simulink library "AEMS_Standard_Library"  (R2016b)
settings: Solver=ode45  StartTime=0.0  StopTime=10.0  RelTol=1e-3
undefined symbols (not defined in the file or in its folder): BkPY, carto, Cbx_extegr, Cbx_lpegrsys, Cbx_portegr, Cnx_bnk_nr_conf, Cnx_cyl_nr_conf, ConfigManagement, configuration_management, Cxx_dcm_io_tmr_end_xxxx, Cxx_dcm_rt_tmr_end, Cxx_DID_xxxx_IO_max, Cxx_DID_xxxx_IO_min, Cxx_egrhsofs, Cxx_vmaniegi, DEM_DEBOUNCE_FREEZE, DEM_DTR_CTL_INVISIBLE, DEM_DTR_CTL_NORMAL, Dem_DtrId2_XXX, Dem_DtrId3_XXX, Dem_DtrId4_XXX, Dem_DtrId5_XXX, Dem_DtrId6_XXX, Dem_DtrId7_XXX, Dem_DtrId8_XXX, Dem_DtrId9_XXX, Dem_DtrId_XXX, Dem_EnableConditionId2_XXX, Dem_EnableConditionId3_XXX, Dem_EnableConditionId4_XXX, Dem_EnableConditionId5_XXX, Dem_EnableConditionId6_XXX, Dem_EnableConditionId7_XXX, Dem_EnableConditionId8_XXX, Dem_EnableConditionId_XXX, Dem_EventId, Dem_EventId2_XXX, Dem_EventId3_XXX, Dem_EventId4_XXX, Dem_EventId5_XXX, Dem_EventId6_XXX, Dem_EventId7_XXX, Dem_EventId8_XXX, Dem_EventId9_XXX, Dem_EventId_Device_Faulttype, Dem_EventId_XXX, DEM_IUMPR_GENERAL_DENOMINATOR, DEM_OPCYC_IGNITION, Dem_RatioId2_XXX, Dem_RatioId3_XXX, Dem_RatioId4_XXX, Dem_RatioId5_XXX, Dem_RatioId6_XXX, Dem_RatioId7_XXX, Dem_RatioId8_XXX, Dem_RatioId_XXX, Dem_StorageConditionId2_XXX, Dem_StorageConditionId3_XXX, Dem_StorageConditionId4_XXX, Dem_StorageConditionId5_XXX ... (+65)
libraries: AEMS_Standard_Library x477, simulink x2
(part 22 of 39)

== system AEMS_Standard_Library/SUB/AEMS_DEM_COUNTER_BASED_DEBOUNCE_THRSHOLD_DYN_6D ==
  note: flag_set
  note: DemDebounceBehavior
  flag_set : Inport
  conditionfulfilled : Inport  Port=2
  prefailed : Inport  Port=3
  prepassed : Inport  Port=4
  failedthreshold : Inport  Port=5
  passedthreshold : Inport  Port=6
  reseteventdebounce : Inport  Port=7
  AEMS_DEM_COUNTER_BASED_DEBOUNCE_THRSHOLD_DYN_CALL1 : Subsystem
  AEMS_DEM_COUNTER_BASED_DEBOUNCE_THRSHOLD_DYN_CALL2 : Subsystem
  AEMS_DEM_COUNTER_BASED_DEBOUNCE_THRSHOLD_DYN_CALL3 : Subsystem
  AEMS_DEM_COUNTER_BASED_DEBOUNCE_THRSHOLD_DYN_CALL4 : Subsystem
  AEMS_DEM_COUNTER_BASED_DEBOUNCE_THRSHOLD_DYN_CALL5 : Subsystem
  AEMS_DEM_COUNTER_BASED_DEBOUNCE_THRSHOLD_DYN_CALL6 : Subsystem
  DemCounterDecrementStepSize : Constant  Value=DemCounterDecrementStepSize
  DemCounterIncrementStepSize : Constant  Value=DemCounterIncrementStepSize
  DemCounterJumpDown : Constant  Value=DemCounterJumpDown
  DemCounterJumpDownValue : Constant  Value=DemCounterJumpDownValue
  DemCounterJumpUp : Constant  Value=DemCounterJumpUp
  DemCounterJumpUpValue : Constant  Value=DemCounterJumpUpValue
  DemDebounceBehavior : Constant  Value=[0,0,0,0,0,0]  OutDataTypeStr=uint8
  Demux{,1..13} (14 alike) : Demux  Outputs=6
  Mux1 : Mux  Inputs=6
  Mux2 : Mux  Inputs=6
  Mux3 : Mux  Inputs=6
  debouncevalue : Outport
  failed : Outport  Port=2
  passed : Outport  Port=3
  wires:
  flag_set/1 -> Demux/1
  Demux/1 -> AEMS_DEM_COUNTER_BASED_DEBOUNCE_THRSHOLD_DYN_CALL1/Enable
  Demux/2 -> AEMS_DEM_COUNTER_BASED_DEBOUNCE_THRSHOLD_DYN_CALL2/Enable
  conditionfulfilled/1 -> Demux1/1  "conditionfulfilled"
  Demux1/1 -> AEMS_DEM_COUNTER_BASED_DEBOUNCE_THRSHOLD_DYN_CALL1/1(conditionfulfilled)
  Demux1/2 -> AEMS_DEM_COUNTER_BASED_DEBOUNCE_THRSHOLD_DYN_CALL2/1(conditionfulfilled)
  prefailed/1 -> Demux2/1  "prefailed"
  Demux2/1 -> AEMS_DEM_COUNTER_BASED_DEBOUNCE_THRSHOLD_DYN_CALL1/2(prefailed)
  Demux2/2 -> AEMS_DEM_COUNTER_BASED_DEBOUNCE_THRSHOLD_DYN_CALL2/2(prefailed)
  prepassed/1 -> Demux3/1  "prepassed"
  Demux3/1 -> AEMS_DEM_COUNTER_BASED_DEBOUNCE_THRSHOLD_DYN_CALL1/3(prepassed)
  Demux3/2 -> AEMS_DEM_COUNTER_BASED_DEBOUNCE_THRSHOLD_DYN_CALL2/3(prepassed)
  DemDebounceBehavior/1 -> Demux4/1  "behavior"
  Demux4/1 -> AEMS_DEM_COUNTER_BASED_DEBOUNCE_THRSHOLD_DYN_CALL1/4(DemDebounceBehavior)
  Demux4/2 -> AEMS_DEM_COUNTER_BASED_DEBOUNCE_THRSHOLD_DYN_CALL2/4(DemDebounceBehavior)
  failedthreshold/1 -> Demux5/1  "failedthreshold"
  Demux5/1 -> AEMS_DEM_COUNTER_BASED_DEBOUNCE_THRSHOLD_DYN_CALL1/5(failedthreshold)
  Demux5/2 -> AEMS_DEM_COUNTER_BASED_DEBOUNCE_THRSHOLD_DYN_CALL2/5(failedthreshold)
  DemCounterIncrementStepSize/1 -> Demux6/1  "incrementstepsize_for_prefailed"
  Demux6/1 -> AEMS_DEM_COUNTER_BASED_DEBOUNCE_THRSHOLD_DYN_CALL1/6(DemCounterIncrementStepSize)
  Demux6/2 -> AEMS_DEM_COUNTER_BASED_DEBOUNCE_THRSHOLD_DYN_CALL2/6(DemCounterIncrementStepSize)
  DemCounterJumpUp/1 -> Demux7/1  "jumpup_activation_with_prefailed"
  Demux7/1 -> AEMS_DEM_COUNTER_BASED_DEBOUNCE_THRSHOLD_DYN_CALL1/7(DemCounterJumpUp)
  Demux7/2 -> AEMS_DEM_COUNTER_BASED_DEBOUNCE_THRSHOLD_DYN_CALL2/7(DemCounterJumpUp)
  DemCounterJumpUpValue/1 -> Demux8/1  "jumpupvalue_with_prefailed"
  Demux8/1 -> AEMS_DEM_COUNTER_BASED_DEBOUNCE_THRSHOLD_DYN_CALL1/8(DemCounterJumpUpValue)
  Demux8/2 -> AEMS_DEM_COUNTER_BASED_DEBOUNCE_THRSHOLD_DYN_CALL2/8(DemCounterJumpUpValue)
  passedthreshold/1 -> Demux9/1  "passedthreshold"
  Demux9/1 -> AEMS_DEM_COUNTER_BASED_DEBOUNCE_THRSHOLD_DYN_CALL1/9(passedthreshold)
  Demux9/2 -> AEMS_DEM_COUNTER_BASED_DEBOUNCE_THRSHOLD_DYN_CALL2/9(passedthreshold)
  DemCounterDecrementStepSize/1 -> Demux10/1  "decrementstepsize_for_prepassed"
  Demux10/1 -> AEMS_DEM_COUNTER_BASED_DEBOUNCE_THRSHOLD_DYN_CALL1/10(DemCounterDecrementStepSize)
  Demux10/2 -> AEMS_DEM_COUNTER_BASED_DEBOUNCE_THRSHOLD_DYN_CALL2/10(DemCounterDecrementStepSize)
  DemCounterJumpDown/1 -> Demux11/1  "jumpdown_activation_with_prepassed"
  Demux11/1 -> AEMS_DEM_COUNTER_BASED_DEBOUNCE_THRSHOLD_DYN_CALL1/11(DemCounterJumpDown)
  Demux11/2 -> AEMS_DEM_COUNTER_BASED_DEBOUNCE_THRSHOLD_DYN_CALL2/11(DemCounterJumpDown)
  DemCounterJumpDownValue/1 -> Demux12/1  "jumpupvalue_with_prefailed"
  Demux12/1 -> AEMS_DEM_COUNTER_BASED_DEBOUNCE_THRSHOLD_DYN_CALL1/12(DemCounterJumpDownValue)
  Demux12/2 -> AEMS_DEM_COUNTER_BASED_DEBOUNCE_THRSHOLD_DYN_CALL2/12(DemCounterJumpDownValue)
  reseteventdebounce/1 -> Demux13/1  "reseteventdebounce"
  Demux13/1 -> AEMS_DEM_COUNTER_BASED_DEBOUNCE_THRSHOLD_DYN_CALL1/13(reseteventdebounce)
  Demux13/2 -> AEMS_DEM_COUNTER_BASED_DEBOUNCE_THRSHOLD_DYN_CALL2/13(reseteventdebounce)
  AEMS_DEM_COUNTER_BASED_DEBOUNCE_THRSHOLD_DYN_CALL1/1(debouncevalue) -> Mux1/1
  Mux1/1 -> debouncevalue/1
  AEMS_DEM_COUNTER_BASED_DEBOUNCE_THRSHOLD_DYN_CALL2/1(debouncevalue) -> Mux1/2
  AEMS_DEM_COUNTER_BASED_DEBOUNCE_THRSHOLD_DYN_CALL1/2(failed) -> Mux2/1
  Mux2/1 -> failed/1
  AEMS_DEM_COUNTER_BASED_DEBOUNCE_THRSHOLD_DYN_CALL2/2(failed) -> Mux2/2
  AEMS_DEM_COUNTER_BASED_DEBOUNCE_THRSHOLD_DYN_CALL1/3(passed) -> Mux3/1
  Mux3/1 -> passed/1
  AEMS_DEM_COUNTER_BASED_DEBOUNCE_THRSHOLD_DYN_CALL2/3(passed) -> Mux3/2
  Demux/3 -> AEMS_DEM_COUNTER_BASED_DEBOUNCE_THRSHOLD_DYN_CALL3/Enable
  Demux1/3 -> AEMS_DEM_COUNTER_BASED_DEBOUNCE_THRSHOLD_DYN_CALL3/1(conditionfulfilled)
  Demux2/3 -> AEMS_DEM_COUNTER_BASED_DEBOUNCE_THRSHOLD_DYN_CALL3/2(prefailed)
  Demux3/3 -> AEMS_DEM_COUNTER_BASED_DEBOUNCE_THRSHOLD_DYN_CALL3/3(prepassed)
  Demux4/3 -> AEMS_DEM_COUNTER_BASED_DEBOUNCE_THRSHOLD_DYN_CALL3/4(DemDebounceBehavior)
  Demux5/3 -> AEMS_DEM_COUNTER_BASED_DEBOUNCE_THRSHOLD_DYN_CALL3/5(failedthreshold)
  Demux6/3 -> AEMS_DEM_COUNTER_BASED_DEBOUNCE_THRSHOLD_DYN_CALL3/6(DemCounterIncrementStepSize)
  Demux7/3 -> AEMS_DEM_COUNTER_BASED_DEBOUNCE_THRSHOLD_DYN_CALL3/7(DemCounterJumpUp)
  Demux8/3 -> AEMS_DEM_COUNTER_BASED_DEBOUNCE_THRSHOLD_DYN_CALL3/8(DemCounterJumpUpValue)
  Demux9/3 -> AEMS_DEM_COUNTER_BASED_DEBOUNCE_THRSHOLD_DYN_CALL3/9(passedthreshold)
  Demux10/3 -> AEMS_DEM_COUNTER_BASED_DEBOUNCE_THRSHOLD_DYN_CALL3/10(DemCounterDecrementStepSize)
  Demux11/3 -> AEMS_DEM_COUNTER_BASED_DEBOUNCE_THRSHOLD_DYN_CALL3/11(DemCounterJumpDown)
  Demux12/3 -> AEMS_DEM_COUNTER_BASED_DEBOUNCE_THRSHOLD_DYN_CALL3/12(DemCounterJumpDownValue)
  Demux13/3 -> AEMS_DEM_COUNTER_BASED_DEBOUNCE_THRSHOLD_DYN_CALL3/13(reseteventdebounce)
  AEMS_DEM_COUNTER_BASED_DEBOUNCE_THRSHOLD_DYN_CALL3/1(debouncevalue) -> Mux1/3
  AEMS_DEM_COUNTER_BASED_DEBOUNCE_THRSHOLD_DYN_CALL3/2(failed) -> Mux2/3
  AEMS_DEM_COUNTER_BASED_DEBOUNCE_THRSHOLD_DYN_CALL3/3(passed) -> Mux3/3
  Demux/4 -> AEMS_DEM_COUNTER_BASED_DEBOUNCE_THRSHOLD_DYN_CALL4/Enable
  Demux/5 -> AEMS_DEM_COUNTER_BASED_DEBOUNCE_THRSHOLD_DYN_CALL5/Enable
  Demux/6 -> AEMS_DEM_COUNTER_BASED_DEBOUNCE_THRSHOLD_DYN_CALL6/Enable
  Demux1/4 -> AEMS_DEM_COUNTER_BASED_DEBOUNCE_THRSHOLD_DYN_CALL4/1(conditionfulfilled)
  Demux1/5 -> AEMS_DEM_COUNTER_BASED_DEBOUNCE_THRSHOLD_DYN_CALL5/1(conditionfulfilled)
  Demux1/6 -> AEMS_DEM_COUNTER_BASED_DEBOUNCE_THRSHOLD_DYN_CALL6/1(conditionfulfilled)
  Demux2/4 -> AEMS_DEM_COUNTER_BASED_DEBOUNCE_THRSHOLD_DYN_CALL4/2(prefailed)
  Demux2/5 -> AEMS_DEM_COUNTER_BASED_DEBOUNCE_THRSHOLD_DYN_CALL5/2(prefailed)
  Demux2/6 -> AEMS_DEM_COUNTER_BASED_DEBOUNCE_THRSHOLD_DYN_CALL6/2(prefailed)
  Demux3/4 -> AEMS_DEM_COUNTER_BASED_DEBOUNCE_THRSHOLD_DYN_CALL4/3(prepassed)
  Demux3/5 -> AEMS_DEM_COUNTER_BASED_DEBOUNCE_THRSHOLD_DYN_CALL5/3(prepassed)
  Demux3/6 -> AEMS_DEM_COUNTER_BASED_DEBOUNCE_THRSHOLD_DYN_CALL6/3(prepassed)
  Demux4/4 -> AEMS_DEM_COUNTER_BASED_DEBOUNCE_THRSHOLD_DYN_CALL4/4(DemDebounceBehavior)
  Demux4/5 -> AEMS_DEM_COUNTER_BASED_DEBOUNCE_THRSHOLD_DYN_CALL5/4(DemDebounceBehavior)
  Demux4/6 -> AEMS_DEM_COUNTER_BASED_DEBOUNCE_THRSHOLD_DYN_CALL6/4(DemDebounceBehavior)
  Demux5/4 -> AEMS_DEM_COUNTER_BASED_DEBOUNCE_THRSHOLD_DYN_CALL4/5(failedthreshold)
  Demux5/5 -> AEMS_DEM_COUNTER_BASED_DEBOUNCE_THRSHOLD_DYN_CALL5/5(failedthreshold)
  Demux5/6 -> AEMS_DEM_COUNTER_BASED_DEBOUNCE_THRSHOLD_DYN_CALL6/5(failedthreshold)
  Demux6/4 -> AEMS_DEM_COUNTER_BASED_DEBOUNCE_THRSHOLD_DYN_CALL4/6(DemCounterIncrementStepSize)
  Demux6/5 -> AEMS_DEM_COUNTER_BASED_DEBOUNCE_THRSHOLD_DYN_CALL5/6(DemCounterIncrementStepSize)
  Demux6/6 -> AEMS_DEM_COUNTER_BASED_DEBOUNCE_THRSHOLD_DYN_CALL6/6(DemCounterIncrementStepSize)
  Demux7/4 -> AEMS_DEM_COUNTER_BASED_DEBOUNCE_THRSHOLD_DYN_CALL4/7(DemCounterJumpUp)
  Demux7/5 -> AEMS_DEM_COUNTER_BASED_DEBOUNCE_THRSHOLD_DYN_CALL5/7(DemCounterJumpUp)
  Demux7/6 -> AEMS_DEM_COUNTER_BASED_DEBOUNCE_THRSHOLD_DYN_CALL6/7(DemCounterJumpUp)
  Demux8/4 -> AEMS_DEM_COUNTER_BASED_DEBOUNCE_THRSHOLD_DYN_CALL4/8(DemCounterJumpUpValue)
  Demux8/5 -> AEMS_DEM_COUNTER_BASED_DEBOUNCE_THRSHOLD_DYN_CALL5/8(DemCounterJumpUpValue)
  Demux8/6 -> AEMS_DEM_COUNTER_BASED_DEBOUNCE_THRSHOLD_DYN_CALL6/8(DemCounterJumpUpValue)
  Demux9/4 -> AEMS_DEM_COUNTER_BASED_DEBOUNCE_THRSHOLD_DYN_CALL4/9(passedthreshold)
  Demux9/5 -> AEMS_DEM_COUNTER_BASED_DEBOUNCE_THRSHOLD_DYN_CALL5/9(passedthreshold)
  Demux9/6 -> AEMS_DEM_COUNTER_BASED_DEBOUNCE_THRSHOLD_DYN_CALL6/9(passedthreshold)
  Demux10/4 -> AEMS_DEM_COUNTER_BASED_DEBOUNCE_THRSHOLD_DYN_CALL4/10(DemCounterDecrementStepSize)
  Demux10/5 -> AEMS_DEM_COUNTER_BASED_DEBOUNCE_THRSHOLD_DYN_CALL5/10(DemCounterDecrementStepSize)
  Demux10/6 -> AEMS_DEM_COUNTER_BASED_DEBOUNCE_THRSHOLD_DYN_CALL6/10(DemCounterDecrementStepSize)
  Demux11/4 -> AEMS_DEM_COUNTER_BASED_DEBOUNCE_THRSHOLD_DYN_CALL4/11(DemCounterJumpDown)
  Demux11/5 -> AEMS_DEM_COUNTER_BASED_DEBOUNCE_THRSHOLD_DYN_CALL5/11(DemCounterJumpDown)
  Demux11/6 -> AEMS_DEM_COUNTER_BASED_DEBOUNCE_THRSHOLD_DYN_CALL6/11(DemCounterJumpDown)
  Demux12/4 -> AEMS_DEM_COUNTER_BASED_DEBOUNCE_THRSHOLD_DYN_CALL4/12(DemCounterJumpDownValue)
  Demux12/5 -> AEMS_DEM_COUNTER_BASED_DEBOUNCE_THRSHOLD_DYN_CALL5/12(DemCounterJumpDownValue)
  Demux12/6 -> AEMS_DEM_COUNTER_BASED_DEBOUNCE_THRSHOLD_DYN_CALL6/12(DemCounterJumpDownValue)
  Demux13/4 -> AEMS_DEM_COUNTER_BASED_DEBOUNCE_THRSHOLD_DYN_CALL4/13(reseteventdebounce)
  Demux13/5 -> AEMS_DEM_COUNTER_BASED_DEBOUNCE_THRSHOLD_DYN_CALL5/13(reseteventdebounce)
  Demux13/6 -> AEMS_DEM_COUNTER_BASED_DEBOUNCE_THRSHOLD_DYN_CALL6/13(reseteventdebounce)
  AEMS_DEM_COUNTER_BASED_DEBOUNCE_THRSHOLD_DYN_CALL4/1(debouncevalue) -> Mux1/4
  AEMS_DEM_COUNTER_BASED_DEBOUNCE_THRSHOLD_DYN_CALL5/1(debouncevalue) -> Mux1/5
  AEMS_DEM_COUNTER_BASED_DEBOUNCE_THRSHOLD_DYN_CALL6/1(debouncevalue) -> Mux1/6
  AEMS_DEM_COUNTER_BASED_DEBOUNCE_THRSHOLD_DYN_CALL4/2(failed) -> Mux2/4
  AEMS_DEM_COUNTER_BASED_DEBOUNCE_THRSHOLD_DYN_CALL5/2(failed) -> Mux2/5
  AEMS_DEM_COUNTER_BASED_DEBOUNCE_THRSHOLD_DYN_CALL6/2(failed) -> Mux2/6
  AEMS_DEM_COUNTER_BASED_DEBOUNCE_THRSHOLD_DYN_CALL4/3(passed) -> Mux3/4
  AEMS_DEM_COUNTER_BASED_DEBOUNCE_THRSHOLD_DYN_CALL5/3(passed) -> Mux3/5
  AEMS_DEM_COUNTER_BASED_DEBOUNCE_THRSHOLD_DYN_CALL6/3(passed) -> Mux3/6

== system AEMS_Standard_Library/SUB/AEMS_DEM_COUNTER_BASED_DEBOUNCE_THRSHOLD_DYN_8D ==
  note: DemDebounceBehavior
  note: flag_set
  flag_set : Inport
  conditionfulfilled : Inport  Port=2
  prefailed : Inport  Port=3
  prepassed : Inport  Port=4
  failedthreshold : Inport  Port=5
  passedthreshold : Inport  Port=6
  reseteventdebounce : Inport  Port=7
  AEMS_DEM_COUNTER_BASED_DEBOUNCE_THRSHOLD_DYN_CALL1 : Subsystem
  AEMS_DEM_COUNTER_BASED_DEBOUNCE_THRSHOLD_DYN_CALL2 : Subsystem
  AEMS_DEM_COUNTER_BASED_DEBOUNCE_THRSHOLD_DYN_CALL3 : Subsystem
  AEMS_DEM_COUNTER_BASED_DEBOUNCE_THRSHOLD_DYN_CALL4 : Subsystem
  AEMS_DEM_COUNTER_BASED_DEBOUNCE_THRSHOLD_DYN_CALL5 : Subsystem
  AEMS_DEM_COUNTER_BASED_DEBOUNCE_THRSHOLD_DYN_CALL6 : Subsystem
  AEMS_DEM_COUNTER_BASED_DEBOUNCE_THRSHOLD_DYN_CALL7 : Subsystem
  AEMS_DEM_COUNTER_BASED_DEBOUNCE_THRSHOLD_DYN_CALL8 : Subsystem
  DemCounterDecrementStepSize : Constant  Value=DemCounterDecrementStepSize
  DemCounterIncrementStepSize : Constant  Value=DemCounterIncrementStepSize
  DemCounterJumpDown : Constant  Value=DemCounterJumpDown
  DemCounterJumpDownValue : Constant  Value=DemCounterJumpDownValue
  DemCounterJumpUp : Constant  Value=DemCounterJumpUp
  DemCounterJumpUpValue : Constant  Value=DemCounterJumpUpValue
  DemDebounceBehavior : Constant  Value=[0,0,0,0,0,0,0,0]  OutDataTypeStr=uint8
  Demux{,1..13} (14 alike) : Demux  Outputs=8
  Mux1 : Mux  Inputs=8
  Mux2 : Mux  Inputs=8
  Mux3 : Mux  Inputs=8
  debouncevalue : Outport
  failed : Outport  Port=2
  passed : Outport  Port=3
  wires:
  AEMS_DEM_COUNTER_BASED_DEBOUNCE_THRSHOLD_DYN_CALL8/3(passed) -> Mux3/8
  AEMS_DEM_COUNTER_BASED_DEBOUNCE_THRSHOLD_DYN_CALL7/3(passed) -> Mux3/7
  AEMS_DEM_COUNTER_BASED_DEBOUNCE_THRSHOLD_DYN_CALL8/2(failed) -> Mux2/8
  AEMS_DEM_COUNTER_BASED_DEBOUNCE_THRSHOLD_DYN_CALL7/2(failed) -> Mux2/7
  AEMS_DEM_COUNTER_BASED_DEBOUNCE_THRSHOLD_DYN_CALL8/1(debouncevalue) -> Mux1/8
  AEMS_DEM_COUNTER_BASED_DEBOUNCE_THRSHOLD_DYN_CALL7/1(debouncevalue) -> Mux1/7
  Demux13/8 -> AEMS_DEM_COUNTER_BASED_DEBOUNCE_THRSHOLD_DYN_CALL8/13(reseteventdebounce)
  Demux13/7 -> AEMS_DEM_COUNTER_BASED_DEBOUNCE_THRSHOLD_DYN_CALL7/13(reseteventdebounce)
  Demux12/8 -> AEMS_DEM_COUNTER_BASED_DEBOUNCE_THRSHOLD_DYN_CALL8/12(DemCounterJumpDownValue)
  Demux12/7 -> AEMS_DEM_COUNTER_BASED_DEBOUNCE_THRSHOLD_DYN_CALL7/12(DemCounterJumpDownValue)
  Demux11/8 -> AEMS_DEM_COUNTER_BASED_DEBOUNCE_THRSHOLD_DYN_CALL8/11(DemCounterJumpDown)
  Demux11/7 -> AEMS_DEM_COUNTER_BASED_DEBOUNCE_THRSHOLD_DYN_CALL7/11(DemCounterJumpDown)
  Demux10/8 -> AEMS_DEM_COUNTER_BASED_DEBOUNCE_THRSHOLD_DYN_CALL8/10(DemCounterDecrementStepSize)
  Demux10/7 -> AEMS_DEM_COUNTER_BASED_DEBOUNCE_THRSHOLD_DYN_CALL7/10(DemCounterDecrementStepSize)
  Demux9/8 -> AEMS_DEM_COUNTER_BASED_DEBOUNCE_THRSHOLD_DYN_CALL8/9(passedthreshold)
  Demux9/7 -> AEMS_DEM_COUNTER_BASED_DEBOUNCE_THRSHOLD_DYN_CALL7/9(passedthreshold)
  Demux8/8 -> AEMS_DEM_COUNTER_BASED_DEBOUNCE_THRSHOLD_DYN_CALL8/8(DemCounterJumpUpValue)
  Demux8/7 -> AEMS_DEM_COUNTER_BASED_DEBOUNCE_THRSHOLD_DYN_CALL7/8(DemCounterJumpUpValue)
  Demux7/8 -> AEMS_DEM_COUNTER_BASED_DEBOUNCE_THRSHOLD_DYN_CALL8/7(DemCounterJumpUp)
  Demux7/7 -> AEMS_DEM_COUNTER_BASED_DEBOUNCE_THRSHOLD_DYN_CALL7/7(DemCounterJumpUp)
  Demux6/8 -> AEMS_DEM_COUNTER_BASED_DEBOUNCE_THRSHOLD_DYN_CALL8/6(DemCounterIncrementStepSize)
  Demux6/7 -> AEMS_DEM_COUNTER_BASED_DEBOUNCE_THRSHOLD_DYN_CALL7/6(DemCounterIncrementStepSize)
  Demux5/8 -> AEMS_DEM_COUNTER_BASED_DEBOUNCE_THRSHOLD_DYN_CALL8/5(failedthreshold)
  Demux5/7 -> AEMS_DEM_COUNTER_BASED_DEBOUNCE_THRSHOLD_DYN_CALL7/5(failedthreshold)
  Demux4/8 -> AEMS_DEM_COUNTER_BASED_DEBOUNCE_THRSHOLD_DYN_CALL8/4(DemDebounceBehavior)
  Demux4/7 -> AEMS_DEM_COUNTER_BASED_DEBOUNCE_THRSHOLD_DYN_CALL7/4(DemDebounceBehavior)
  Demux3/8 -> AEMS_DEM_COUNTER_BASED_DEBOUNCE_THRSHOLD_DYN_CALL8/3(prepassed)
  Demux3/7 -> AEMS_DEM_COUNTER_BASED_DEBOUNCE_THRSHOLD_DYN_CALL7/3(prepassed)
  Demux2/8 -> AEMS_DEM_COUNTER_BASED_DEBOUNCE_THRSHOLD_DYN_CALL8/2(prefailed)
  Demux2/7 -> AEMS_DEM_COUNTER_BASED_DEBOUNCE_THRSHOLD_DYN_CALL7/2(prefailed)
  Demux1/8 -> AEMS_DEM_COUNTER_BASED_DEBOUNCE_THRSHOLD_DYN_CALL8/1(conditionfulfilled)
  Demux1/7 -> AEMS_DEM_COUNTER_BASED_DEBOUNCE_THRSHOLD_DYN_CALL7/1(conditionfulfilled)
  Demux/8 -> AEMS_DEM_COUNTER_BASED_DEBOUNCE_THRSHOLD_DYN_CALL8/Enable
  Demux/7 -> AEMS_DEM_COUNTER_BASED_DEBOUNCE_THRSHOLD_DYN_CALL7/Enable
  AEMS_DEM_COUNTER_BASED_DEBOUNCE_THRSHOLD_DYN_CALL6/3(passed) -> Mux3/6
  AEMS_DEM_COUNTER_BASED_DEBOUNCE_THRSHOLD_DYN_CALL5/3(passed) -> Mux3/5
  AEMS_DEM_COUNTER_BASED_DEBOUNCE_THRSHOLD_DYN_CALL4/3(passed) -> Mux3/4
  AEMS_DEM_COUNTER_BASED_DEBOUNCE_THRSHOLD_DYN_CALL6/2(failed) -> Mux2/6
  AEMS_DEM_COUNTER_BASED_DEBOUNCE_THRSHOLD_DYN_CALL5/2(failed) -> Mux2/5
  AEMS_DEM_COUNTER_BASED_DEBOUNCE_THRSHOLD_DYN_CALL4/2(failed) -> Mux2/4
  AEMS_DEM_COUNTER_BASED_DEBOUNCE_THRSHOLD_DYN_CALL6/1(debouncevalue) -> Mux1/6
  AEMS_DEM_COUNTER_BASED_DEBOUNCE_THRSHOLD_DYN_CALL5/1(debouncevalue) -> Mux1/5
  AEMS_DEM_COUNTER_BASED_DEBOUNCE_THRSHOLD_DYN_CALL4/1(debouncevalue) -> Mux1/4
  Demux13/6 -> AEMS_DEM_COUNTER_BASED_DEBOUNCE_THRSHOLD_DYN_CALL6/13(reseteventdebounce)
  Demux13/5 -> AEMS_DEM_COUNTER_BASED_DEBOUNCE_THRSHOLD_DYN_CALL5/13(reseteventdebounce)
  Demux13/4 -> AEMS_DEM_COUNTER_BASED_DEBOUNCE_THRSHOLD_DYN_CALL4/13(reseteventdebounce)
  Demux12/6 -> AEMS_DEM_COUNTER_BASED_DEBOUNCE_THRSHOLD_DYN_CALL6/12(DemCounterJumpDownValue)
  Demux12/5 -> AEMS_DEM_COUNTER_BASED_DEBOUNCE_THRSHOLD_DYN_CALL5/12(DemCounterJumpDownValue)
  Demux12/4 -> AEMS_DEM_COUNTER_BASED_DEBOUNCE_THRSHOLD_DYN_CALL4/12(DemCounterJumpDownValue)
  Demux11/6 -> AEMS_DEM_COUNTER_BASED_DEBOUNCE_THRSHOLD_DYN_CALL6/11(DemCounterJumpDown)
  Demux11/5 -> AEMS_DEM_COUNTER_BASED_DEBOUNCE_THRSHOLD_DYN_CALL5/11(DemCounterJumpDown)
  Demux11/4 -> AEMS_DEM_COUNTER_BASED_DEBOUNCE_THRSHOLD_DYN_CALL4/11(DemCounterJumpDown)
  Demux10/6 -> AEMS_DEM_COUNTER_BASED_DEBOUNCE_THRSHOLD_DYN_CALL6/10(DemCounterDecrementStepSize)
  Demux10/5 -> AEMS_DEM_COUNTER_BASED_DEBOUNCE_THRSHOLD_DYN_CALL5/10(DemCounterDecrementStepSize)
  Demux10/4 -> AEMS_DEM_COUNTER_BASED_DEBOUNCE_THRSHOLD_DYN_CALL4/10(DemCounterDecrementStepSize)
  Demux9/6 -> AEMS_DEM_COUNTER_BASED_DEBOUNCE_THRSHOLD_DYN_CALL6/9(passedthreshold)
  Demux9/5 -> AEMS_DEM_COUNTER_BASED_DEBOUNCE_THRSHOLD_DYN_CALL5/9(passedthreshold)
  Demux9/4 -> AEMS_DEM_COUNTER_BASED_DEBOUNCE_THRSHOLD_DYN_CALL4/9(passedthreshold)
  Demux8/6 -> AEMS_DEM_COUNTER_BASED_DEBOUNCE_THRSHOLD_DYN_CALL6/8(DemCounterJumpUpValue)
  Demux8/5 -> AEMS_DEM_COUNTER_BASED_DEBOUNCE_THRSHOLD_DYN_CALL5/8(DemCounterJumpUpValue)
  Demux8/4 -> AEMS_DEM_COUNTER_BASED_DEBOUNCE_THRSHOLD_DYN_CALL4/8(DemCounterJumpUpValue)
  Demux7/6 -> AEMS_DEM_COUNTER_BASED_DEBOUNCE_THRSHOLD_DYN_CALL6/7(DemCounterJumpUp)
  Demux7/5 -> AEMS_DEM_COUNTER_BASED_DEBOUNCE_THRSHOLD_DYN_CALL5/7(DemCounterJumpUp)
  Demux7/4 -> AEMS_DEM_COUNTER_BASED_DEBOUNCE_THRSHOLD_DYN_CALL4/7(DemCounterJumpUp)
  Demux6/6 -> AEMS_DEM_COUNTER_BASED_DEBOUNCE_THRSHOLD_DYN_CALL6/6(DemCounterIncrementStepSize)
  Demux6/5 -> AEMS_DEM_COUNTER_BASED_DEBOUNCE_THRSHOLD_DYN_CALL5/6(DemCounterIncrementStepSize)
  Demux6/4 -> AEMS_DEM_COUNTER_BASED_DEBOUNCE_THRSHOLD_DYN_CALL4/6(DemCounterIncrementStepSize)
  Demux5/6 -> AEMS_DEM_COUNTER_BASED_DEBOUNCE_THRSHOLD_DYN_CALL6/5(failedthreshold)
  Demux5/5 -> AEMS_DEM_COUNTER_BASED_DEBOUNCE_THRSHOLD_DYN_CALL5/5(failedthreshold)
  Demux5/4 -> AEMS_DEM_COUNTER_BASED_DEBOUNCE_THRSHOLD_DYN_CALL4/5(failedthreshold)
  Demux4/6 -> AEMS_DEM_COUNTER_BASED_DEBOUNCE_THRSHOLD_DYN_CALL6/4(DemDebounceBehavior)
  Demux4/5 -> AEMS_DEM_COUNTER_BASED_DEBOUNCE_THRSHOLD_DYN_CALL5/4(DemDebounceBehavior)
  Demux4/4 -> AEMS_DEM_COUNTER_BASED_DEBOUNCE_THRSHOLD_DYN_CALL4/4(DemDebounceBehavior)
  Demux3/6 -> AEMS_DEM_COUNTER_BASED_DEBOUNCE_THRSHOLD_DYN_CALL6/3(prepassed)
  Demux3/5 -> AEMS_DEM_COUNTER_BASED_DEBOUNCE_THRSHOLD_DYN_CALL5/3(prepassed)
  Demux3/4 -> AEMS_DEM_COUNTER_BASED_DEBOUNCE_THRSHOLD_DYN_CALL4/3(prepassed)
  Demux2/6 -> AEMS_DEM_COUNTER_BASED_DEBOUNCE_THRSHOLD_DYN_CALL6/2(prefailed)
  Demux2/5 -> AEMS_DEM_COUNTER_BASED_DEBOUNCE_THRSHOLD_DYN_CALL5/2(prefailed)
  Demux2/4 -> AEMS_DEM_COUNTER_BASED_DEBOUNCE_THRSHOLD_DYN_CALL4/2(prefailed)
  Demux1/6 -> AEMS_DEM_COUNTER_BASED_DEBOUNCE_THRSHOLD_DYN_CALL6/1(conditionfulfilled)
  Demux1/5 -> AEMS_DEM_COUNTER_BASED_DEBOUNCE_THRSHOLD_DYN_CALL5/1(conditionfulfilled)
  Demux1/4 -> AEMS_DEM_COUNTER_BASED_DEBOUNCE_THRSHOLD_DYN_CALL4/1(conditionfulfilled)
  Demux/6 -> AEMS_DEM_COUNTER_BASED_DEBOUNCE_THRSHOLD_DYN_CALL6/Enable
  Demux/5 -> AEMS_DEM_COUNTER_BASED_DEBOUNCE_THRSHOLD_DYN_CALL5/Enable
  Demux/4 -> AEMS_DEM_COUNTER_BASED_DEBOUNCE_THRSHOLD_DYN_CALL4/Enable
  AEMS_DEM_COUNTER_BASED_DEBOUNCE_THRSHOLD_DYN_CALL3/3(passed) -> Mux3/3
  AEMS_DEM_COUNTER_BASED_DEBOUNCE_THRSHOLD_DYN_CALL3/2(failed) -> Mux2/3
  AEMS_DEM_COUNTER_BASED_DEBOUNCE_THRSHOLD_DYN_CALL3/1(debouncevalue) -> Mux1/3
  Demux13/3 -> AEMS_DEM_COUNTER_BASED_DEBOUNCE_THRSHOLD_DYN_CALL3/13(reseteventdebounce)
  Demux12/3 -> AEMS_DEM_COUNTER_BASED_DEBOUNCE_THRSHOLD_DYN_CALL3/12(DemCounterJumpDownValue)
  Demux11/3 -> AEMS_DEM_COUNTER_BASED_DEBOUNCE_THRSHOLD_DYN_CALL3/11(DemCounterJumpDown)
  Demux10/3 -> AEMS_DEM_COUNTER_BASED_DEBOUNCE_THRSHOLD_DYN_CALL3/10(DemCounterDecrementStepSize)
  Demux9/3 -> AEMS_DEM_COUNTER_BASED_DEBOUNCE_THRSHOLD_DYN_CALL3/9(passedthreshold)
  Demux8/3 -> AEMS_DEM_COUNTER_BASED_DEBOUNCE_THRSHOLD_DYN_CALL3/8(DemCounterJumpUpValue)
  Demux7/3 -> AEMS_DEM_COUNTER_BASED_DEBOUNCE_THRSHOLD_DYN_CALL3/7(DemCounterJumpUp)
  Demux6/3 -> AEMS_DEM_COUNTER_BASED_DEBOUNCE_THRSHOLD_DYN_CALL3/6(DemCounterIncrementStepSize)
  Demux5/3 -> AEMS_DEM_COUNTER_BASED_DEBOUNCE_THRSHOLD_DYN_CALL3/5(failedthreshold)
  Demux4/3 -> AEMS_DEM_COUNTER_BASED_DEBOUNCE_THRSHOLD_DYN_CALL3/4(DemDebounceBehavior)
  Demux3/3 -> AEMS_DEM_COUNTER_BASED_DEBOUNCE_THRSHOLD_DYN_CALL3/3(prepassed)
  Demux2/3 -> AEMS_DEM_COUNTER_BASED_DEBOUNCE_THRSHOLD_DYN_CALL3/2(prefailed)
  Demux1/3 -> AEMS_DEM_COUNTER_BASED_DEBOUNCE_THRSHOLD_DYN_CALL3/1(conditionfulfilled)
  Demux/3 -> AEMS_DEM_COUNTER_BASED_DEBOUNCE_THRSHOLD_DYN_CALL3/Enable
  AEMS_DEM_COUNTER_BASED_DEBOUNCE_THRSHOLD_DYN_CALL2/3(passed) -> Mux3/2
  Mux3/1 -> passed/1
  AEMS_DEM_COUNTER_BASED_DEBOUNCE_THRSHOLD_DYN_CALL1/3(passed) -> Mux3/1
  AEMS_DEM_COUNTER_BASED_DEBOUNCE_THRSHOLD_DYN_CALL2/2(failed) -> Mux2/2
  Mux2/1 -> failed/1
  AEMS_DEM_COUNTER_BASED_DEBOUNCE_THRSHOLD_DYN_CALL1/2(failed) -> Mux2/1
  AEMS_DEM_COUNTER_BASED_DEBOUNCE_THRSHOLD_DYN_CALL2/1(debouncevalue) -> Mux1/2
  Mux1/1 -> debouncevalue/1
  AEMS_DEM_COUNTER_BASED_DEBOUNCE_THRSHOLD_DYN_CALL1/1(debouncevalue) -> Mux1/1
  Demux13/2 -> AEMS_DEM_COUNTER_BASED_DEBOUNCE_THRSHOLD_DYN_CALL2/13(reseteventdebounce)
  Demux13/1 -> AEMS_DEM_COUNTER_BASED_DEBOUNCE_THRSHOLD_DYN_CALL1/13(reseteventdebounce)
  reseteventdebounce/1 -> Demux13/1  "reseteventdebounce"
  Demux12/2 -> AEMS_DEM_COUNTER_BASED_DEBOUNCE_THRSHOLD_DYN_CALL2/12(DemCounterJumpDownValue)
  Demux12/1 -> AEMS_DEM_COUNTER_BASED_DEBOUNCE_THRSHOLD_DYN_CALL1/12(DemCounterJumpDownValue)
  DemCounterJumpDownValue/1 -> Demux12/1  "jumpupvalue_with_prefailed"
  Demux11/2 -> AEMS_DEM_COUNTER_BASED_DEBOUNCE_THRSHOLD_DYN_CALL2/11(DemCounterJumpDown)
  Demux11/1 -> AEMS_DEM_COUNTER_BASED_DEBOUNCE_THRSHOLD_DYN_CALL1/11(DemCounterJumpDown)
  DemCounterJumpDown/1 -> Demux11/1  "jumpdown_activation_with_prepassed"
  Demux10/2 -> AEMS_DEM_COUNTER_BASED_DEBOUNCE_THRSHOLD_DYN_CALL2/10(DemCounterDecrementStepSize)
  Demux10/1 -> AEMS_DEM_COUNTER_BASED_DEBOUNCE_THRSHOLD_DYN_CALL1/10(DemCounterDecrementStepSize)
  DemCounterDecrementStepSize/1 -> Demux10/1  "decrementstepsize_for_prepassed"
  Demux9/2 -> AEMS_DEM_COUNTER_BASED_DEBOUNCE_THRSHOLD_DYN_CALL2/9(passedthreshold)
  Demux9/1 -> AEMS_DEM_COUNTER_BASED_DEBOUNCE_THRSHOLD_DYN_CALL1/9(passedthreshold)
  passedthreshold/1 -> Demux9/1  "passedthreshold"
  Demux8/2 -> AEMS_DEM_COUNTER_BASED_DEBOUNCE_THRSHOLD_DYN_CALL2/8(DemCounterJumpUpValue)
  Demux8/1 -> AEMS_DEM_COUNTER_BASED_DEBOUNCE_THRSHOLD_DYN_CALL1/8(DemCounterJumpUpValue)
  DemCounterJumpUpValue/1 -> Demux8/1  "jumpupvalue_with_prefailed"
  Demux7/2 -> AEMS_DEM_COUNTER_BASED_DEBOUNCE_THRSHOLD_DYN_CALL2/7(DemCounterJumpUp)
  Demux7/1 -> AEMS_DEM_COUNTER_BASED_DEBOUNCE_THRSHOLD_DYN_CALL1/7(DemCounterJumpUp)
  DemCounterJumpUp/1 -> Demux7/1  "jumpup_activation_with_prefailed"
  Demux6/2 -> AEMS_DEM_COUNTER_BASED_DEBOUNCE_THRSHOLD_DYN_CALL2/6(DemCounterIncrementStepSize)
  Demux6/1 -> AEMS_DEM_COUNTER_BASED_DEBOUNCE_THRSHOLD_DYN_CALL1/6(DemCounterIncrementStepSize)
  DemCounterIncrementStepSize/1 -> Demux6/1  "incrementstepsize_for_prefailed"
  Demux5/2 -> AEMS_DEM_COUNTER_BASED_DEBOUNCE_THRSHOLD_DYN_CALL2/5(failedthreshold)
  Demux5/1 -> AEMS_DEM_COUNTER_BASED_DEBOUNCE_THRSHOLD_DYN_CALL1/5(failedthreshold)
  failedthreshold/1 -> Demux5/1  "failedthreshold"
  Demux4/2 -> AEMS_DEM_COUNTER_BASED_DEBOUNCE_THRSHOLD_DYN_CALL2/4(DemDebounceBehavior)
  Demux4/1 -> AEMS_DEM_COUNTER_BASED_DEBOUNCE_THRSHOLD_DYN_CALL1/4(DemDebounceBehavior)
  DemDebounceBehavior/1 -> Demux4/1  "behavior"
  Demux3/2 -> AEMS_DEM_COUNTER_BASED_DEBOUNCE_THRSHOLD_DYN_CALL2/3(prepassed)
  Demux3/1 -> AEMS_DEM_COUNTER_BASED_DEBOUNCE_THRSHOLD_DYN_CALL1/3(prepassed)
  prepassed/1 -> Demux3/1  "prepassed"
  Demux2/2 -> AEMS_DEM_COUNTER_BASED_DEBOUNCE_THRSHOLD_DYN_CALL2/2(prefailed)
  Demux2/1 -> AEMS_DEM_COUNTER_BASED_DEBOUNCE_THRSHOLD_DYN_CALL1/2(prefailed)
  prefailed/1 -> Demux2/1  "prefailed"
  Demux1/2 -> AEMS_DEM_COUNTER_BASED_DEBOUNCE_THRSHOLD_DYN_CALL2/1(conditionfulfilled)
  Demux1/1 -> AEMS_DEM_COUNTER_BASED_DEBOUNCE_THRSHOLD_DYN_CALL1/1(conditionfulfilled)
  conditionfulfilled/1 -> Demux1/1  "conditionfulfilled"
  Demux/2 -> AEMS_DEM_COUNTER_BASED_DEBOUNCE_THRSHOLD_DYN_CALL2/Enable
  Demux/1 -> AEMS_DEM_COUNTER_BASED_DEBOUNCE_THRSHOLD_DYN_CALL1/Enable
  flag_set/1 -> Demux/1

== system AEMS_Standard_Library/SUB/AEMS_DEM_GETEVENTSTATUS ==
  eventid : Inport
  Data Type Conversion : DataTypeConversion  OutDataTypeStr=uint8  SaturateOnIntegerOverflow=on
  Data Type Conversion1 : DataTypeConversion  OutDataTypeStr=uint8
  Ground1 : Ground
  Source_Of_Permission_Port : Ground
  Terminator : Terminator
  Terminator1 : Terminator
  eventstatusextended : Outport
  wires:
  Source_Of_Permission_Port/1 -> Data Type Conversion/1
  Data Type Conversion/1 -> eventstatusextended/1  "eventstatusextended"
  eventid/1 -> Terminator/1
  Ground1/1 -> Data Type Conversion1/1
  Data Type Conversion1/1 -> Terminator1/1  "Std_ReturnType"

== system AEMS_Standard_Library/SUB/AEMS_DEM_GETINDICATORSTATUS ==
  indicator_id : Inport
  Data Type Conversion : DataTypeConversion  OutDataTypeStr=uint8  SaturateOnIntegerOverflow=on
  Data Type Conversion1 : DataTypeConversion  OutDataTypeStr=uint8
  Ground1 : Ground
  Source_Of_Permission_Port : Constant  Value=0  OutDataTypeStr=Inherit: Inherit via back propagation
  Terminator : Terminator
  Terminator1 : Terminator
  indicator_status : Outport
  wires:
  Data Type Conversion/1 -> indicator_status/1  "indicator_status"
  Source_Of_Permission_Port/1 -> Data Type Conversion/1
  indicator_id/1 -> Terminator/1  "indicator_id"
  Ground1/1 -> Data Type Conversion1/1
  Data Type Conversion1/1 -> Terminator1/1  "Std_ReturnType"

== system AEMS_Standard_Library/SUB/AEMS_DEM_GET_EVENT_STS_1D ==
  AEMS_DEM_GETEVENTSTATUS : AEMS_Standard_Library/SUB/AEMS_DEM_GETEVENTSTATUS  Tag=[LIB]  EventId=Dem_EventId_XXX  FunctionMode=Dysfunctional
      settings: AttributesFormatString=%<MaskType>\nFunction Mode : = %<FunctionMode>
  AEMS_DEM_LIB_BIT_EXTRACT : AEMS_Standard_Library/SUB/AEMS_DEM_LIB_BIT_EXTRACT  Tag=[LIB]  extract_bit=132
      settings: AttributesFormatString=%<MaskType>\nextract_bit = %<extract_bit>
  EventId_Block : Constant  Value=Dem_EventId_XXX  OutDataTypeStr=uint16
  diag_status_flag : Outport
  wires:
  AEMS_DEM_GETEVENTSTATUS/1 -> AEMS_DEM_LIB_BIT_EXTRACT/1
  EventId_Block/1 -> AEMS_DEM_GETEVENTSTATUS/1
  AEMS_DEM_LIB_BIT_EXTRACT/1 -> diag_status_flag/1  "diag_status_flag"

== system AEMS_Standard_Library/SUB/AEMS_DEM_GET_EVENT_STS_2D ==
  AEMS_DEM_GETEVENTSTATUS : AEMS_Standard_Library/SUB/AEMS_DEM_GETEVENTSTATUS  Tag=[LIB]  EventId=Dem_EventId_XXX  FunctionMode=Dysfunctional
      settings: AttributesFormatString=%<MaskType>\nFunction Mode : = %<FunctionMode>
  AEMS_DEM_GETEVENTSTATUS1 : AEMS_Standard_Library/SUB/AEMS_DEM_GETEVENTSTATUS  Tag=[LIB]  EventId=Dem_EventId2_XXX  FunctionMode=Dysfunctional
      settings: AttributesFormatString=%<MaskType>\nFunction Mode : = %<FunctionMode>
  DEM_LIB_BIT_EXTRACT1 : AEMS_Standard_Library/SUB/AEMS_DEM_LIB_BIT_EXTRACT  Tag=[LIB]  extract_bit=132
      settings: AttributesFormatString=%<MaskType>\nextract_bit = %<extract_bit>
  DEM_LIB_BIT_EXTRACT2 : AEMS_Standard_Library/SUB/AEMS_DEM_LIB_BIT_EXTRACT  Tag=[LIB]  extract_bit=132
      settings: AttributesFormatString=%<MaskType>\nextract_bit = %<extract_bit>
  Data Type Conversion : DataTypeConversion  OutDataTypeStr=boolean  SaturateOnIntegerOverflow=on
  EventId_Block1 : Constant  Value=Dem_EventId_XXX  OutDataTypeStr=uint16
  EventId_Block2 : Constant  Value=Dem_EventId2_XXX  OutDataTypeStr=uint16
  Mux : Mux  Inputs=2
  diag_status_flag : Outport
  wires:
  EventId_Block1/1 -> AEMS_DEM_GETEVENTSTATUS/1
  DEM_LIB_BIT_EXTRACT1/1 -> Mux/1  "diag_status_flag1"
  EventId_Block2/1 -> AEMS_DEM_GETEVENTSTATUS1/1
  DEM_LIB_BIT_EXTRACT2/1 -> Mux/2  "diag_status_flag2"
  Mux/1 -> Data Type Conversion/1
  Data Type Conversion/1 -> diag_status_flag/1  "diag_status_flag"
  AEMS_DEM_GETEVENTSTATUS/1 -> DEM_LIB_BIT_EXTRACT1/1
  AEMS_DEM_GETEVENTSTATUS1/1 -> DEM_LIB_BIT_EXTRACT2/1

== system AEMS_Standard_Library/SUB/AEMS_DEM_GET_EVENT_STS_8D ==
  AEMS_DEM_GETEVENTSTATUS1 : AEMS_Standard_Library/SUB/AEMS_DEM_GETEVENTSTATUS  Tag=[LIB]  EventId=Dem_EventId_XXX  FunctionMode=Dysfunctional
      settings: AttributesFormatString=%<MaskType>\nFunction Mode : = %<FunctionMode>
  AEMS_DEM_GETEVENTSTATUS2 : AEMS_Standard_Library/SUB/AEMS_DEM_GETEVENTSTATUS  Tag=[LIB]  EventId=Dem_EventId2_XXX  FunctionMode=Dysfunctional
      settings: AttributesFormatString=%<MaskType>\nFunction Mode : = %<FunctionMode>
  AEMS_DEM_GETEVENTSTATUS3 : AEMS_Standard_Library/SUB/AEMS_DEM_GETEVENTSTATUS  Tag=[LIB]  EventId=Dem_EventId3_XXX  FunctionMode=Dysfunctional
      settings: AttributesFormatString=%<MaskType>\nFunction Mode : = %<FunctionMode>
  AEMS_DEM_GETEVENTSTATUS4 : AEMS_Standard_Library/SUB/AEMS_DEM_GETEVENTSTATUS  Tag=[LIB]  EventId=Dem_EventId4_XXX  FunctionMode=Dysfunctional
      settings: AttributesFormatString=%<MaskType>\nFunction Mode : = %<FunctionMode>
  AEMS_DEM_GETEVENTSTATUS5 : AEMS_Standard_Library/SUB/AEMS_DEM_GETEVENTSTATUS  Tag=[LIB]  EventId=Dem_EventId5_XXX  FunctionMode=Dysfunctional
      settings: AttributesFormatString=%<MaskType>\nFunction Mode : = %<FunctionMode>
  AEMS_DEM_GETEVENTSTATUS6 : AEMS_Standard_Library/SUB/AEMS_DEM_GETEVENTSTATUS  Tag=[LIB]  EventId=Dem_EventId6_XXX  FunctionMode=Dysfunctional
      settings: AttributesFormatString=%<MaskType>\nFunction Mode : = %<FunctionMode>
  AEMS_DEM_GETEVENTSTATUS7 : AEMS_Standard_Library/SUB/AEMS_DEM_GETEVENTSTATUS  Tag=[LIB]  EventId=Dem_EventId7_XXX  FunctionMode=Dysfunctional
      settings: AttributesFormatString=%<MaskType>\nFunction Mode : = %<FunctionMode>
  AEMS_DEM_GETEVENTSTATUS8 : AEMS_Standard_Library/SUB/AEMS_DEM_GETEVENTSTATUS  Tag=[LIB]  EventId=Dem_EventId8_XXX  FunctionMode=Dysfunctional
      settings: AttributesFormatString=%<MaskType>\nFunction Mode : = %<FunctionMode>
  DEM_LIB_BIT_EXTRACT{1..8} (8 alike) : AEMS_Standard_Library/SUB/AEMS_DEM_LIB_BIT_EXTRACT  Tag=[LIB]  extract_bit=132
      settings: AttributesFormatString=%<MaskType>\nextract_bit = %<extract_bit>
  Data Type Conversion : DataTypeConversion  OutDataTypeStr=boolean  SaturateOnIntegerOverflow=on
  EventId_Block1 : Constant  Value=Dem_EventId_XXX  OutDataTypeStr=uint16
  EventId_Block2 : Constant  Value=Dem_EventId2_XXX  OutDataTypeStr=uint16
  EventId_Block3 : Constant  Value=Dem_EventId3_XXX  OutDataTypeStr=uint16
  EventId_Block4 : Constant  Value=Dem_EventId4_XXX  OutDataTypeStr=uint16
  EventId_Block5 : Constant  Value=Dem_EventId5_XXX  OutDataTypeStr=uint16
  EventId_Block6 : Constant  Value=Dem_EventId6_XXX  OutDataTypeStr=uint16
  EventId_Block7 : Constant  Value=Dem_EventId7_XXX  OutDataTypeStr=uint16
  EventId_Block8 : Constant  Value=Dem_EventId8_XXX  OutDataTypeStr=uint16
  Mux : Mux  Inputs=8
  diag_status_flag : Outport
  wires:
  Mux/1 -> Data Type Conversion/1
  DEM_LIB_BIT_EXTRACT2/1 -> Mux/2  "diag_status_flag2"
  EventId_Block2/1 -> AEMS_DEM_GETEVENTSTATUS2/1
  DEM_LIB_BIT_EXTRACT1/1 -> Mux/1  "diag_status_flag1"
  EventId_Block1/1 -> AEMS_DEM_GETEVENTSTATUS1/1
  DEM_LIB_BIT_EXTRACT3/1 -> Mux/3  "diag_status_flag3"
  EventId_Block3/1 -> AEMS_DEM_GETEVENTSTATUS3/1
  DEM_LIB_BIT_EXTRACT4/1 -> Mux/4  "diag_status_flag4"
  EventId_Block4/1 -> AEMS_DEM_GETEVENTSTATUS4/1
  DEM_LIB_BIT_EXTRACT5/1 -> Mux/5  "diag_status_flag5"
  EventId_Block5/1 -> AEMS_DEM_GETEVENTSTATUS5/1
  DEM_LIB_BIT_EXTRACT6/1 -> Mux/6  "diag_status_flag6"
  EventId_Block6/1 -> AEMS_DEM_GETEVENTSTATUS6/1
  DEM_LIB_BIT_EXTRACT7/1 -> Mux/7  "diag_status_flag7"
  EventId_Block7/1 -> AEMS_DEM_GETEVENTSTATUS7/1
  DEM_LIB_BIT_EXTRACT8/1 -> Mux/8  "diag_status_flag8"
  EventId_Block8/1 -> AEMS_DEM_GETEVENTSTATUS8/1
  Data Type Conversion/1 -> diag_status_flag/1  "diag_status_flag"
  AEMS_DEM_GETEVENTSTATUS1/1 -> DEM_LIB_BIT_EXTRACT1/1
  AEMS_DEM_GETEVENTSTATUS2/1 -> DEM_LIB_BIT_EXTRACT2/1
  AEMS_DEM_GETEVENTSTATUS3/1 -> DEM_LIB_BIT_EXTRACT3/1
  AEMS_DEM_GETEVENTSTATUS4/1 -> DEM_LIB_BIT_EXTRACT4/1
  AEMS_DEM_GETEVENTSTATUS5/1 -> DEM_LIB_BIT_EXTRACT5/1
  AEMS_DEM_GETEVENTSTATUS6/1 -> DEM_LIB_BIT_EXTRACT6/1
  AEMS_DEM_GETEVENTSTATUS7/1 -> DEM_LIB_BIT_EXTRACT7/1
  AEMS_DEM_GETEVENTSTATUS8/1 -> DEM_LIB_BIT_EXTRACT8/1

== system AEMS_Standard_Library/SUB/AEMS_DEM_GET_EVENT_STS_9D ==
  AEMS_DEM_GETEVENTSTATUS1 : AEMS_Standard_Library/SUB/AEMS_DEM_GETEVENTSTATUS  Tag=[LIB]  EventId=Dem_EventId_XXX  FunctionMode=Dysfunctional
      settings: AttributesFormatString=%<MaskType>\nFunction Mode : = %<FunctionMode>
  AEMS_DEM_GETEVENTSTATUS2 : AEMS_Standard_Library/SUB/AEMS_DEM_GETEVENTSTATUS  Tag=[LIB]  EventId=Dem_EventId2_XXX  FunctionMode=Dysfunctional
      settings: AttributesFormatString=%<MaskType>\nFunction Mode : = %<FunctionMode>
  AEMS_DEM_GETEVENTSTATUS3 : AEMS_Standard_Library/SUB/AEMS_DEM_GETEVENTSTATUS  Tag=[LIB]  EventId=Dem_EventId3_XXX  FunctionMode=Dysfunctional
      settings: AttributesFormatString=%<MaskType>\nFunction Mode : = %<FunctionMode>
  AEMS_DEM_GETEVENTSTATUS4 : AEMS_Standard_Library/SUB/AEMS_DEM_GETEVENTSTATUS  Tag=[LIB]  EventId=Dem_EventId4_XXX  FunctionMode=Dysfunctional
      settings: AttributesFormatString=%<MaskType>\nFunction Mode : = %<FunctionMode>
  AEMS_DEM_GETEVENTSTATUS5 : AEMS_Standard_Library/SUB/AEMS_DEM_GETEVENTSTATUS  Tag=[LIB]  EventId=Dem_EventId5_XXX  FunctionMode=Dysfunctional
      settings: AttributesFormatString=%<MaskType>\nFunction Mode : = %<FunctionMode>
  AEMS_DEM_GETEVENTSTATUS6 : AEMS_Standard_Library/SUB/AEMS_DEM_GETEVENTSTATUS  Tag=[LIB]  EventId=Dem_EventId6_XXX  FunctionMode=Dysfunctional
      settings: AttributesFormatString=%<MaskType>\nFunction Mode : = %<FunctionMode>
  AEMS_DEM_GETEVENTSTATUS7 : AEMS_Standard_Library/SUB/AEMS_DEM_GETEVENTSTATUS  Tag=[LIB]  EventId=Dem_EventId7_XXX  FunctionMode=Dysfunctional
      settings: AttributesFormatString=%<MaskType>\nFunction Mode : = %<FunctionMode>
  AEMS_DEM_GETEVENTSTATUS8 : AEMS_Standard_Library/SUB/AEMS_DEM_GETEVENTSTATUS  Tag=[LIB]  EventId=Dem_EventId8_XXX  FunctionMode=Dysfunctional
      settings: AttributesFormatString=%<MaskType>\nFunction Mode : = %<FunctionMode>
  AEMS_DEM_GETEVENTSTATUS9 : AEMS_Standard_Library/SUB/AEMS_DEM_GETEVENTSTATUS  Tag=[LIB]  EventId=Dem_EventId9_XXX  FunctionMode=Dysfunctional
      settings: AttributesFormatString=%<MaskType>\nFunction Mode : = %<FunctionMode>
  DEM_LIB_BIT_EXTRACT{1..9} (9 alike) : AEMS_Standard_Library/SUB/AEMS_DEM_LIB_BIT_EXTRACT  Tag=[LIB]  extract_bit=132
      settings: AttributesFormatString=%<MaskType>\nextract_bit = %<extract_bit>
  Data Type Conversion : DataTypeConversion  OutDataTypeStr=boolean  SaturateOnIntegerOverflow=on
  EventId_Block0 : Constant  Value=Dem_EventId_XXX  OutDataTypeStr=uint16
  EventId_Block1 : Constant  Value=Dem_EventId2_XXX  OutDataTypeStr=uint16
  EventId_Block2 : Constant  Value=Dem_EventId3_XXX  OutDataTypeStr=uint16
  EventId_Block3 : Constant  Value=Dem_EventId4_XXX  OutDataTypeStr=uint16
  EventId_Block4 : Constant  Value=Dem_EventId5_XXX  OutDataTypeStr=uint16
  EventId_Block5 : Constant  Value=Dem_EventId6_XXX  OutDataTypeStr=uint16
  EventId_Block6 : Constant  Value=Dem_EventId7_XXX  OutDataTypeStr=uint16
  EventId_Block7 : Constant  Value=Dem_EventId8_XXX  OutDataTypeStr=uint16
  EventId_Block8 : Constant  Value=Dem_EventId9_XXX  OutDataTypeStr=uint16
  Mux : Mux  Inputs=9
  diag_status_flag : Outport
  wires:
  DEM_LIB_BIT_EXTRACT9/1 -> Mux/9  "diag_status_flag8"
  DEM_LIB_BIT_EXTRACT8/1 -> Mux/8  "diag_status_flag7"
  DEM_LIB_BIT_EXTRACT7/1 -> Mux/7  "diag_status_flag6"
  DEM_LIB_BIT_EXTRACT6/1 -> Mux/6  "diag_status_flag5"
  DEM_LIB_BIT_EXTRACT5/1 -> Mux/5  "diag_status_flag4"
  DEM_LIB_BIT_EXTRACT4/1 -> Mux/4  "diag_status_flag3"
  DEM_LIB_BIT_EXTRACT3/1 -> Mux/3  "diag_status_flag2"
  DEM_LIB_BIT_EXTRACT2/1 -> Mux/2  "diag_status_flag1"
  DEM_LIB_BIT_EXTRACT1/1 -> Mux/1  "diag_status_flag0"
  EventId_Block0/1 -> AEMS_DEM_GETEVENTSTATUS1/1
  AEMS_DEM_GETEVENTSTATUS1/1 -> DEM_LIB_BIT_EXTRACT1/1
  Mux/1 -> Data Type Conversion/1
  EventId_Block2/1 -> AEMS_DEM_GETEVENTSTATUS3/1
  EventId_Block1/1 -> AEMS_DEM_GETEVENTSTATUS2/1
  EventId_Block3/1 -> AEMS_DEM_GETEVENTSTATUS4/1
  EventId_Block4/1 -> AEMS_DEM_GETEVENTSTATUS5/1
  EventId_Block5/1 -> AEMS_DEM_GETEVENTSTATUS6/1
  EventId_Block6/1 -> AEMS_DEM_GETEVENTSTATUS7/1
  EventId_Block7/1 -> AEMS_DEM_GETEVENTSTATUS8/1
  EventId_Block8/1 -> AEMS_DEM_GETEVENTSTATUS9/1
  Data Type Conversion/1 -> diag_status_flag/1  "diag_status_flag"
  AEMS_DEM_GETEVENTSTATUS2/1 -> DEM_LIB_BIT_EXTRACT2/1
  AEMS_DEM_GETEVENTSTATUS3/1 -> DEM_LIB_BIT_EXTRACT3/1
  AEMS_DEM_GETEVENTSTATUS4/1 -> DEM_LIB_BIT_EXTRACT4/1
  AEMS_DEM_GETEVENTSTATUS5/1 -> DEM_LIB_BIT_EXTRACT5/1
  AEMS_DEM_GETEVENTSTATUS6/1 -> DEM_LIB_BIT_EXTRACT6/1
  AEMS_DEM_GETEVENTSTATUS7/1 -> DEM_LIB_BIT_EXTRACT7/1
  AEMS_DEM_GETEVENTSTATUS8/1 -> DEM_LIB_BIT_EXTRACT8/1
  AEMS_DEM_GETEVENTSTATUS9/1 -> DEM_LIB_BIT_EXTRACT9/1

== system AEMS_Standard_Library/SUB/AEMS_DEM_LIB_BIT_EXTRACT ==
  integer_input : Inport
  AEMS_BITWISEAND : AEMS_Standard_Library/BIT_OPERATION/AEMS_BITWISEAND  Tag=[LIB]
      settings: AttributesFormatString=%<MaskType>
  RelationalOperator1 : RelationalOperator  Operator=>  OutDataTypeStr=boolean  RndMeth=Nearest  InputSameDT=on
  bit_check : Constant  Value=4  OutDataTypeStr=uint8
  bit_diff : Constant  Value=0  OutDataTypeStr=uint8
  bit_check_result : Outport
  wires:
  RelationalOperator1/1 -> bit_check_result/1  "bit_check_result"
  bit_diff/1 -> RelationalOperator1/2
  bit_check/1 -> AEMS_BITWISEAND/2
  integer_input/1 -> AEMS_BITWISEAND/1  "integer_input"
  AEMS_BITWISEAND/1 -> RelationalOperator1/1

== system AEMS_Standard_Library/SUB/AEMS_DEM_LIB_BIT_EXTRACT_FDGNOK ==
  integer_input : Inport
  AEMS_BITWISEAND : AEMS_Standard_Library/BIT_OPERATION/AEMS_BITWISEAND  Tag=[LIB]
      settings: AttributesFormatString=%<MaskType>
  AEMS_BITWISEAND1 : AEMS_Standard_Library/BIT_OPERATION/AEMS_BITWISEAND  Tag=[LIB]
      settings: AttributesFormatString=%<MaskType>
  RelationalOperator1 : RelationalOperator  Operator=>  OutDataTypeStr=boolean  RndMeth=Nearest  InputSameDT=on
  RelationalOperator2 : RelationalOperator  Operator=>  OutDataTypeStr=boolean  RndMeth=Nearest  InputSameDT=on
  bit_check1 : Constant  Value=2  OutDataTypeStr=uint8
  bit_check2 : Constant  Value=64  OutDataTypeStr=uint8
  bit_diff1 : Constant  Value=0  OutDataTypeStr=uint8
  bit_diff2 : Constant  Value=0  OutDataTypeStr=uint8
  extract_logic : Logic  OutDataTypeStr=boolean
  extract_logic1 : Logic  Operator=NOT  OutDataTypeStr=boolean
  extract_logic2 : Logic  Operator=NOT  OutDataTypeStr=boolean
  bit_check_result : Outport
  wires:
  RelationalOperator2/1 -> extract_logic2/1
  RelationalOperator1/1 -> extract_logic1/1
  bit_diff2/1 -> RelationalOperator2/2
  bit_check2/1 -> AEMS_BITWISEAND1/2
  AEMS_BITWISEAND1/1 -> RelationalOperator2/1
  bit_diff1/1 -> RelationalOperator1/2
  bit_check1/1 -> AEMS_BITWISEAND/2
  integer_input/1 -> AEMS_BITWISEAND/1, AEMS_BITWISEAND1/1  "integer_input"
  AEMS_BITWISEAND/1 -> RelationalOperator1/1
  extract_logic/1 -> bit_check_result/1  "bit_check_result"
  extract_logic1/1 -> extract_logic/1
  extract_logic2/1 -> extract_logic/2

== system AEMS_Standard_Library/SUB/AEMS_DEM_LIB_BIT_EXTRACT_FS_RESET ==
  integer_input : Inport
  AEMS_BITWISEAND : AEMS_Standard_Library/BIT_OPERATION/AEMS_BITWISEAND  Tag=[LIB]
      settings: AttributesFormatString=%<MaskType>
  AEMS_BITWISEAND1 : AEMS_Standard_Library/BIT_OPERATION/AEMS_BITWISEAND  Tag=[LIB]
      settings: AttributesFormatString=%<MaskType>
  RelationalOperator1 : RelationalOperator  Operator=>  OutDataTypeStr=boolean  RndMeth=Nearest  InputSameDT=on
  RelationalOperator2 : RelationalOperator  Operator=>  OutDataTypeStr=boolean  RndMeth=Nearest  InputSameDT=on
  bit_check1 : Constant  OutDataTypeStr=uint8
  bit_check2 : Constant  Value=64  OutDataTypeStr=uint8
  bit_diff1 : Constant  Value=0  OutDataTypeStr=uint8
  bit_diff2 : Constant  Value=0  OutDataTypeStr=uint8
  extract_logic : Logic  OutDataTypeStr=boolean
  extract_logic1 : Logic  Operator=NOT  OutDataTypeStr=boolean
  bit_check_result : Outport
  wires:
  RelationalOperator2/1 -> extract_logic1/1
  RelationalOperator1/1 -> extract_logic/1
  bit_diff2/1 -> RelationalOperator2/2
  bit_check2/1 -> AEMS_BITWISEAND1/2
  AEMS_BITWISEAND1/1 -> RelationalOperator2/1
  bit_diff1/1 -> RelationalOperator1/2
  bit_check1/1 -> AEMS_BITWISEAND/2
  integer_input/1 -> AEMS_BITWISEAND/1, AEMS_BITWISEAND1/1  "integer_input"
  AEMS_BITWISEAND/1 -> RelationalOperator1/1
  extract_logic/1 -> bit_check_result/1  "bit_check_result"
  extract_logic1/1 -> extract_logic/2

== system AEMS_Standard_Library/SUB/AEMS_DEM_READDATAOFPID01 ==
  Data Type Conversion{1..5} (5 alike) : DataTypeConversion  OutDataTypeStr=uint8  SaturateOnIntegerOverflow=on
  Data Type Conversion6 : DataTypeConversion  OutDataTypeStr=uint8
  Ground{,1..4} (5 alike) : Ground
  Mux : Mux
  Terminator1 : Terminator
  vPID01 : Outport
  wires:
  Data Type Conversion4/1 -> vPID01/1
  Ground3/1 -> Data Type Conversion5/1  "dummy_4"
  Ground2/1 -> Data Type Conversion3/1  "dummy_3"
  Ground1/1 -> Data Type Conversion2/1  "dummy_2"
  Ground/1 -> Data Type Conversion1/1  "dummy_1"
  Mux/1 -> Data Type Conversion4/1
  Data Type Conversion1/1 -> Mux/1
  Data Type Conversion2/1 -> Mux/2
  Data Type Conversion3/1 -> Mux/3
  Data Type Conversion5/1 -> Mux/4
  Ground4/1 -> Data Type Conversion6/1
  Data Type Conversion6/1 -> Terminator1/1  "Std_ReturnType"

== system AEMS_Standard_Library/SUB/AEMS_DEM_REPIUMPRDENLOCK ==
  ratioid : Inport
  Data Type Conversion1 : DataTypeConversion  OutDataTypeStr=uint8
  Ground1 : Ground
  Terminator : Terminator
  Terminator1 : Terminator
  wires:
  ratioid/1 -> Terminator/1  "ratioid"
  Ground1/1 -> Data Type Conversion1/1
  Data Type Conversion1/1 -> Terminator1/1  "Std_ReturnType"

== system AEMS_Standard_Library/SUB/AEMS_DEM_REPIUMPRDENRELEASE ==
  ratioid : Inport
  Data Type Conversion1 : DataTypeConversion  OutDataTypeStr=uint8
  Ground1 : Ground
  Terminator : Terminator
  Terminator1 : Terminator
  wires:
  ratioid/1 -> Terminator/1  "ratioid"
  Ground1/1 -> Data Type Conversion1/1
  Data Type Conversion1/1 -> Terminator1/1  "Std_ReturnType"

== system AEMS_Standard_Library/SUB/AEMS_DEM_REPIUMPRFAULTDETECT ==
  ratioid : Inport
  Data Type Conversion1 : DataTypeConversion  OutDataTypeStr=uint8
  Ground1 : Ground
  Terminator : Terminator
  Terminator1 : Terminator
  wires:
  ratioid/1 -> Terminator/1  "ratioid"
  Ground1/1 -> Data Type Conversion1/1
  Data Type Conversion1/1 -> Terminator1/1  "Std_ReturnType"

== system AEMS_Standard_Library/SUB/AEMS_DEM_REP_IUMPR_1D ==
  denlock_status : Inport  OutDataTypeStr=boolean  PortDimensions=1
  faultdetect_trigger : Inport  Port=2  OutDataTypeStr=boolean  PortDimensions=1
  AEMS_EDGE_FALLING : AEMS_Standard_Library/EDGE/AEMS_EDGE_FALLING  Tag=[LIB]  init=false
      settings: AttributesFormatString=|
      | %<MaskType>
      | Initial Value : %<init>
  AEMS_EDGE_RISING : AEMS_Standard_Library/EDGE/AEMS_EDGE_RISING  Tag=[LIB]  init=false
      settings: AttributesFormatString=|
      | %<MaskType>
      | Initial Value : %<init>
  AEMS_EDGE_RISING1 : AEMS_Standard_Library/EDGE/AEMS_EDGE_RISING  Tag=[LIB]  init=false
      settings: AttributesFormatString=|
      | %<MaskType>
      | Initial Value : %<init>
  Dem_RepIUMPRDenLock_call1 : Subsystem  TreatAsAtomicUnit=on
  Dem_RepIUMPRDenRelease_call1 : Subsystem  TreatAsAtomicUnit=on
  Dem_RepIUMPRFaultDetect_call1 : Subsystem  TreatAsAtomicUnit=on
  wires:
  faultdetect_trigger/1 -> AEMS_EDGE_RISING/1  "faultdetect_trigger"
  denlock_status/1 -> AEMS_EDGE_RISING1/1, AEMS_EDGE_FALLING/1  "denlock_status"
  AEMS_EDGE_RISING/1 -> Dem_RepIUMPRFaultDetect_call1/Enable  "faultdetect_call1"
  AEMS_EDGE_RISING1/1 -> Dem_RepIUMPRDenLock_call1/Enable  "denlock_call1"
  AEMS_EDGE_FALLING/1 -> Dem_RepIUMPRDenRelease_call1/Enable  "denrelease_call1"

== system AEMS_Standard_Library/SUB/AEMS_DEM_REP_IUMPR_2D ==
  denlock_status : Inport
  faultdetect_trigger : Inport  Port=2
  AEMS_EDGE_FALLING : AEMS_Standard_Library/EDGE/AEMS_EDGE_FALLING  Tag=[LIB]  init=false
      settings: AttributesFormatString=|
      | %<MaskType>
      | Initial Value : %<init>
  AEMS_EDGE_RISING1 : AEMS_Standard_Library/EDGE/AEMS_EDGE_RISING  Tag=[LIB]  init=false
      settings: AttributesFormatString=|
      | %<MaskType>
      | Initial Value : %<init>
  AEMS_EDGE_RISING2 : AEMS_Standard_Library/EDGE/AEMS_EDGE_RISING  Tag=[LIB]  init=false
      settings: AttributesFormatString=|
      | %<MaskType>
      | Initial Value : %<init>
  Dem_RepIUMPRDenLock_Call1 : Subsystem  TreatAsAtomicUnit=on
  Dem_RepIUMPRDenLock_Call2 : Subsystem  TreatAsAtomicUnit=on
  Dem_RepIUMPRDenRelease_Call1 : Subsystem  TreatAsAtomicUnit=on
  Dem_RepIUMPRDenRelease_Call2 : Subsystem  TreatAsAtomicUnit=on
  Dem_RepIUMPRFaultDetect_Call1 : Subsystem  TreatAsAtomicUnit=on
  Dem_RepIUMPRFaultDetect_Call2 : Subsystem  TreatAsAtomicUnit=on
  Demux : Demux  Outputs=2
  Demux1 : Demux  Outputs=2
  Demux2 : Demux  Outputs=2
  wires:
  Demux1/2 -> Dem_RepIUMPRDenLock_Call2/Enable  "denlock_call2"
  Demux1/1 -> Dem_RepIUMPRDenLock_Call1/Enable  "denlock_call1"
  AEMS_EDGE_FALLING/1 -> Demux2/1  "denrelease_call"
  Demux2/2 -> Dem_RepIUMPRDenRelease_Call2/Enable  "denrelease_call2"
  Demux2/1 -> Dem_RepIUMPRDenRelease_Call1/Enable  "denrelease_call1"
  AEMS_EDGE_RISING2/1 -> Demux1/1  "denlock_call"
  Demux/2 -> Dem_RepIUMPRFaultDetect_Call2/Enable  "faultdetect_call2"
  Demux/1 -> Dem_RepIUMPRFaultDetect_Call1/Enable  "faultdetect_call1"
  AEMS_EDGE_RISING1/1 -> Demux/1  "faultdetect_call"
  faultdetect_trigger/1 -> AEMS_EDGE_RISING1/1  "faultdetect_trigger"
  denlock_status/1 -> AEMS_EDGE_RISING2/1, AEMS_EDGE_FALLING/1  "denlock_status"
